simulink model "test_mdl_NI"  (R2018a)
settings: Solver=VariableStepAuto  StartTime=0.0  StopTime=10.0  RelTol=1e-3
(part 11 of 24)

== system test_mdl_NI/Subsystem/IPMA_ADAS/AutoDriveBeam_Data2_Ox3C1 ==
  in_port : Inport
  AdbBrdr2CritLeft_T_Stat : Terminator
  AdbBrdr2CritRigh_T_Stat : Terminator
  AdbBrdr2DistLeft_D_Stat : Terminator
  AdbBrdr2DistRigh_D_Stat : Terminator
  AdbBrdr2Left_An_Rq : Terminator
  AdbBrdr2Low_An_Rq : Terminator
  AdbBrdr2Right_An_Rq : Terminator
  AdbBrdr2Up_An_Rq : Terminator
  AdbIntns2_D_Rq : Terminator
  AdbMde2_D_Rq : Terminator
  bus_selector : BusSelector  OutputSignals=AdbBrdr2CritLeft_T_Stat,AdbBrdr2CritRigh_T_Stat,AdbBrdr2DistLeft_D_Stat,AdbBrdr2DistRigh_D_Stat,AdbBrdr2Left_An_Rq,AdbBrdr2Low_An_Rq,AdbBrdr2Right_An_Rq,AdbBrdr2Up_An_Rq,AdbIntns2_D_Rq,AdbMde2_D_Rq
  wires:
  in_port/1 -> bus_selector/1  "AutoDriveBeam_Data2_Ox3C1"
  bus_selector/1 -> AdbBrdr2CritLeft_T_Stat/1  "<AdbBrdr2CritLeft_T_Stat>"
  bus_selector/2 -> AdbBrdr2CritRigh_T_Stat/1  "<AdbBrdr2CritRigh_T_Stat>"
  bus_selector/3 -> AdbBrdr2DistLeft_D_Stat/1  "<AdbBrdr2DistLeft_D_Stat>"
  bus_selector/4 -> AdbBrdr2DistRigh_D_Stat/1  "<AdbBrdr2DistRigh_D_Stat>"
  bus_selector/5 -> AdbBrdr2Left_An_Rq/1  "<AdbBrdr2Left_An_Rq>"
  bus_selector/6 -> AdbBrdr2Low_An_Rq/1  "<AdbBrdr2Low_An_Rq>"
  bus_selector/7 -> AdbBrdr2Right_An_Rq/1  "<AdbBrdr2Right_An_Rq>"
  bus_selector/8 -> AdbBrdr2Up_An_Rq/1  "<AdbBrdr2Up_An_Rq>"
  bus_selector/9 -> AdbIntns2_D_Rq/1  "<AdbIntns2_D_Rq>"
  bus_selector/10 -> AdbMde2_D_Rq/1  "<AdbMde2_D_Rq>"

== system test_mdl_NI/Subsystem/IPMA_ADAS/AutoDriveBeam_Data3_Ox3C2 ==
  in_port : Inport
  AdbBrdr3CritLeft_T_Stat : Terminator
  AdbBrdr3CritRigh_T_Stat : Terminator
  AdbBrdr3DistLeft_D_Stat : Terminator
  AdbBrdr3DistRigh_D_Stat : Terminator
  AdbBrdr3Left_An_Rq : Terminator
  AdbBrdr3Low_An_Rq : Terminator
  AdbBrdr3Right_An_Rq : Terminator
  AdbBrdr3Up_An_Rq : Terminator
  AdbIntns3_D_Rq : Terminator
  AdbMde3_D_Rq : Terminator
  bus_selector : BusSelector  OutputSignals=AdbBrdr3CritLeft_T_Stat,AdbBrdr3CritRigh_T_Stat,AdbBrdr3DistLeft_D_Stat,AdbBrdr3DistRigh_D_Stat,AdbBrdr3Left_An_Rq,AdbBrdr3Low_An_Rq,AdbBrdr3Right_An_Rq,AdbBrdr3Up_An_Rq,AdbIntns3_D_Rq,AdbMde3_D_Rq
  wires:
  in_port/1 -> bus_selector/1  "AutoDriveBeam_Data3_Ox3C2"
  bus_selector/1 -> AdbBrdr3CritLeft_T_Stat/1  "<AdbBrdr3CritLeft_T_Stat>"
  bus_selector/2 -> AdbBrdr3CritRigh_T_Stat/1  "<AdbBrdr3CritRigh_T_Stat>"
  bus_selector/3 -> AdbBrdr3DistLeft_D_Stat/1  "<AdbBrdr3DistLeft_D_Stat>"
  bus_selector/4 -> AdbBrdr3DistRigh_D_Stat/1  "<AdbBrdr3DistRigh_D_Stat>"
  bus_selector/5 -> AdbBrdr3Left_An_Rq/1  "<AdbBrdr3Left_An_Rq>"
  bus_selector/6 -> AdbBrdr3Low_An_Rq/1  "<AdbBrdr3Low_An_Rq>"
  bus_selector/7 -> AdbBrdr3Right_An_Rq/1  "<AdbBrdr3Right_An_Rq>"
  bus_selector/8 -> AdbBrdr3Up_An_Rq/1  "<AdbBrdr3Up_An_Rq>"
  bus_selector/9 -> AdbIntns3_D_Rq/1  "<AdbIntns3_D_Rq>"
  bus_selector/10 -> AdbMde3_D_Rq/1  "<AdbMde3_D_Rq>"

== system test_mdl_NI/Subsystem/IPMA_ADAS/Bndry_Alert_L_Data_Ox3A1 ==
  in_port : Inport
  BalrChimeLeft_D_Rq : Terminator
  BalrLckLeft_B_Stat : Terminator
  BalrLeft_D_Stat : Terminator
  BalrMdeLeft_D_Stat : Terminator
  BalrMdeSelLeft_B_Stat : Terminator
  BalrSnsLeft_D_Falt : Terminator
  BalrWndwLeft_B_Stat : Terminator
  CamraRearOn_B_RqBalrl : Terminator
  DrLckActv_B_RqBalrl : Terminator
  DrLckCnt_No_ActlBalrl : Terminator
  WndwDrvRear_D_RqBalrl : Terminator
  WndwDrv_D_RqBalrl : Terminator
  WndwPsngrRear_D_RqBalrl : Terminator
  WndwPsngr_D_RqBalrl : Terminator
  bus_selector : BusSelector  OutputSignals=BalrChimeLeft_D_Rq,BalrLckLeft_B_Stat,BalrLeft_D_Stat,BalrMdeLeft_D_Stat,BalrMdeSelLeft_B_Stat,BalrSnsLeft_D_Falt,BalrWndwLeft_B_Stat,CamraRearOn_B_RqBalrl,DrLckActv_B_RqBalrl,DrLckCnt_No_ActlBalrl,WndwDrvRear_D_RqBalrl,WndwDrv_D_RqBalrl,WndwPsngrRear_D_RqBalrl,WndwPsngr_D_RqBalrl
  wires:
  in_port/1 -> bus_selector/1  "Bndry_Alert_L_Data_Ox3A1"
  bus_selector/1 -> BalrChimeLeft_D_Rq/1  "<BalrChimeLeft_D_Rq>"
  bus_selector/2 -> BalrLckLeft_B_Stat/1  "<BalrLckLeft_B_Stat>"
  bus_selector/3 -> BalrLeft_D_Stat/1  "<BalrLeft_D_Stat>"
  bus_selector/4 -> BalrMdeLeft_D_Stat/1  "<BalrMdeLeft_D_Stat>"
  bus_selector/5 -> BalrMdeSelLeft_B_Stat/1  "<BalrMdeSelLeft_B_Stat>"
  bus_selector/6 -> BalrSnsLeft_D_Falt/1  "<BalrSnsLeft_D_Falt>"
  bus_selector/7 -> BalrWndwLeft_B_Stat/1  "<BalrWndwLeft_B_Stat>"
  bus_selector/8 -> CamraRearOn_B_RqBalrl/1  "<CamraRearOn_B_RqBalrl>"
  bus_selector/9 -> DrLckActv_B_RqBalrl/1  "<DrLckActv_B_RqBalrl>"
  bus_selector/10 -> DrLckCnt_No_ActlBalrl/1  "<DrLckCnt_No_ActlBalrl>"
  bus_selector/11 -> WndwDrvRear_D_RqBalrl/1  "<WndwDrvRear_D_RqBalrl>"
  bus_selector/12 -> WndwDrv_D_RqBalrl/1  "<WndwDrv_D_RqBalrl>"
  bus_selector/13 -> WndwPsngrRear_D_RqBalrl/1  "<WndwPsngrRear_D_RqBalrl>"
  bus_selector/14 -> WndwPsngr_D_RqBalrl/1  "<WndwPsngr_D_RqBalrl>"

== system test_mdl_NI/Subsystem/IPMA_ADAS/Bndry_Alert_R_Data_Ox3A2 ==
  in_port : Inport
  BalrChimeRight_D_Rq : Terminator
  BalrLckRight_B_Stat : Terminator
  BalrMdeRight_D_Stat : Terminator
  BalrMdeSelRight_B_Stat : Terminator
  BalrRight_D_Stat : Terminator
  BalrSnsRight_D_Falt : Terminator
  BalrWndwRight_B_Stat : Terminator
  CamraRearOn_B_RqBalrr : Terminator
  DrLckActv_B_RqBalrr : Terminator
  DrLckCnt_No_ActlBalrr : Terminator
  WndwDrvRear_D_RqBalrr : Terminator
  WndwDrv_D_RqBalrr : Terminator
  WndwPsngrRear_D_RqBalrr : Terminator
  WndwPsngr_D_RqBalrr : Terminator
  bus_selector : BusSelector  OutputSignals=BalrChimeRight_D_Rq,BalrLckRight_B_Stat,BalrMdeRight_D_Stat,BalrMdeSelRight_B_Stat,BalrRight_D_Stat,BalrSnsRight_D_Falt,BalrWndwRight_B_Stat,CamraRearOn_B_RqBalrr,DrLckActv_B_RqBalrr,DrLckCnt_No_ActlBalrr,WndwDrvRear_D_RqBalrr,WndwDrv_D_RqBalrr,WndwPsngrRear_D_RqBalrr,WndwPsngr_D_RqBalrr
  wires:
  in_port/1 -> bus_selector/1  "Bndry_Alert_R_Data_Ox3A2"
  bus_selector/1 -> BalrChimeRight_D_Rq/1  "<BalrChimeRight_D_Rq>"
  bus_selector/2 -> BalrLckRight_B_Stat/1  "<BalrLckRight_B_Stat>"
  bus_selector/3 -> BalrMdeRight_D_Stat/1  "<BalrMdeRight_D_Stat>"
  bus_selector/4 -> BalrMdeSelRight_B_Stat/1  "<BalrMdeSelRight_B_Stat>"
  bus_selector/5 -> BalrRight_D_Stat/1  "<BalrRight_D_Stat>"
  bus_selector/6 -> BalrSnsRight_D_Falt/1  "<BalrSnsRight_D_Falt>"
  bus_selector/7 -> BalrWndwRight_B_Stat/1  "<BalrWndwRight_B_Stat>"
  bus_selector/8 -> CamraRearOn_B_RqBalrr/1  "<CamraRearOn_B_RqBalrr>"
  bus_selector/9 -> DrLckActv_B_RqBalrr/1  "<DrLckActv_B_RqBalrr>"
  bus_selector/10 -> DrLckCnt_No_ActlBalrr/1  "<DrLckCnt_No_ActlBalrr>"
  bus_selector/11 -> WndwDrvRear_D_RqBalrr/1  "<WndwDrvRear_D_RqBalrr>"
  bus_selector/12 -> WndwDrv_D_RqBalrr/1  "<WndwDrv_D_RqBalrr>"
  bus_selector/13 -> WndwPsngrRear_D_RqBalrr/1  "<WndwPsngrRear_D_RqBalrr>"
  bus_selector/14 -> WndwPsngr_D_RqBalrr/1  "<WndwPsngr_D_RqBalrr>"

== system test_mdl_NI/Subsystem/IPMA_ADAS/BoundaryAlert_Left_1_Ox4E0 ==
  in_port : Inport
  BalrLeft1CurntX_L_Actl : Terminator
  BalrLeft1CurntY_L_Actl : Terminator
  BalrLeft1Dsply_B_Stat : Terminator
  BalrLeft1Fast_B_Stat : Terminator
  BalrLeft1Prev1X_L_Actl : Terminator
  BalrLeft1Prev1Y_L_Actl : Terminator
  BalrLeft1Prev2X_L_Actl : Terminator
  BalrLeft1Prev2Y_L_Actl : Terminator
  BalrLeft1Prev3X_L_Actl : Terminator
  BalrLeft1Prev3Y_L_Actl : Terminator
  BalrLeft1Threat_D_Stat : Terminator
  bus_selector : BusSelector  OutputSignals=BalrLeft1CurntX_L_Actl,BalrLeft1CurntY_L_Actl,BalrLeft1Dsply_B_Stat,BalrLeft1Fast_B_Stat,BalrLeft1Prev1X_L_Actl,BalrLeft1Prev1Y_L_Actl,BalrLeft1Prev2X_L_Actl,BalrLeft1Prev2Y_L_Actl,BalrLeft1Prev3X_L_Actl,BalrLeft1Prev3Y_L_Actl,BalrLeft1Threat_D_Stat
  wires:
  in_port/1 -> bus_selector/1  "BoundaryAlert_Left_1_Ox4E0"
  bus_selector/1 -> BalrLeft1CurntX_L_Actl/1  "<BalrLeft1CurntX_L_Actl>"
  bus_selector/2 -> BalrLeft1CurntY_L_Actl/1  "<BalrLeft1CurntY_L_Actl>"
  bus_selector/3 -> BalrLeft1Dsply_B_Stat/1  "<BalrLeft1Dsply_B_Stat>"
  bus_selector/4 -> BalrLeft1Fast_B_Stat/1  "<BalrLeft1Fast_B_Stat>"
  bus_selector/5 -> BalrLeft1Prev1X_L_Actl/1  "<BalrLeft1Prev1X_L_Actl>"
  bus_selector/6 -> BalrLeft1Prev1Y_L_Actl/1  "<BalrLeft1Prev1Y_L_Actl>"
  bus_selector/7 -> BalrLeft1Prev2X_L_Actl/1  "<BalrLeft1Prev2X_L_Actl>"
  bus_selector/8 -> BalrLeft1Prev2Y_L_Actl/1  "<BalrLeft1Prev2Y_L_Actl>"
  bus_selector/9 -> BalrLeft1Prev3X_L_Actl/1  "<BalrLeft1Prev3X_L_Actl>"
  bus_selector/10 -> BalrLeft1Prev3Y_L_Actl/1  "<BalrLeft1Prev3Y_L_Actl>"
  bus_selector/11 -> BalrLeft1Threat_D_Stat/1  "<BalrLeft1Threat_D_Stat>"

== system test_mdl_NI/Subsystem/IPMA_ADAS/BoundaryAlert_Left_2_Ox4E1 ==
  in_port : Inport
  BalrLeft2CurntX_L_Actl : Terminator
  BalrLeft2CurntY_L_Actl : Terminator
  BalrLeft2Dsply_B_Stat : Terminator
  BalrLeft2Fast_B_Stat : Terminator
  BalrLeft2Prev1X_L_Actl : Terminator
  BalrLeft2Prev1Y_L_Actl : Terminator
  BalrLeft2Prev2X_L_Actl : Terminator
  BalrLeft2Prev2Y_L_Actl : Terminator
  BalrLeft2Prev3X_L_Actl : Terminator
  BalrLeft2Prev3Y_L_Actl : Terminator
  BalrLeft2Threat_D_Stat : Terminator
  bus_selector : BusSelector  OutputSignals=BalrLeft2CurntX_L_Actl,BalrLeft2CurntY_L_Actl,BalrLeft2Dsply_B_Stat,BalrLeft2Fast_B_Stat,BalrLeft2Prev1X_L_Actl,BalrLeft2Prev1Y_L_Actl,BalrLeft2Prev2X_L_Actl,BalrLeft2Prev2Y_L_Actl,BalrLeft2Prev3X_L_Actl,BalrLeft2Prev3Y_L_Actl,BalrLeft2Threat_D_Stat
  wires:
  in_port/1 -> bus_selector/1  "BoundaryAlert_Left_2_Ox4E1"
  bus_selector/1 -> BalrLeft2CurntX_L_Actl/1  "<BalrLeft2CurntX_L_Actl>"
  bus_selector/2 -> BalrLeft2CurntY_L_Actl/1  "<BalrLeft2CurntY_L_Actl>"
  bus_selector/3 -> BalrLeft2Dsply_B_Stat/1  "<BalrLeft2Dsply_B_Stat>"
  bus_selector/4 -> BalrLeft2Fast_B_Stat/1  "<BalrLeft2Fast_B_Stat>"
  bus_selector/5 -> BalrLeft2Prev1X_L_Actl/1  "<BalrLeft2Prev1X_L_Actl>"
  bus_selector/6 -> BalrLeft2Prev1Y_L_Actl/1  "<BalrLeft2Prev1Y_L_Actl>"
  bus_selector/7 -> BalrLeft2Prev2X_L_Actl/1  "<BalrLeft2Prev2X_L_Actl>"
  bus_selector/8 -> BalrLeft2Prev2Y_L_Actl/1  "<BalrLeft2Prev2Y_L_Actl>"
  bus_selector/9 -> BalrLeft2Prev3X_L_Actl/1  "<BalrLeft2Prev3X_L_Actl>"
  bus_selector/10 -> BalrLeft2Prev3Y_L_Actl/1  "<BalrLeft2Prev3Y_L_Actl>"
  bus_selector/11 -> BalrLeft2Threat_D_Stat/1  "<BalrLeft2Threat_D_Stat>"

== system test_mdl_NI/Subsystem/IPMA_ADAS/BoundaryAlert_Left_3_Ox4E2 ==
  in_port : Inport
  BalrLeft3CurntX_L_Actl : Terminator
  BalrLeft3CurntY_L_Actl : Terminator
  BalrLeft3Dsply_B_Stat : Terminator
  BalrLeft3Fast_B_Stat : Terminator
  BalrLeft3Prev1X_L_Actl : Terminator
  BalrLeft3Prev1Y_L_Actl : Terminator
  BalrLeft3Prev2X_L_Actl : Terminator
  BalrLeft3Prev2Y_L_Actl : Terminator
  BalrLeft3Prev3X_L_Actl : Terminator
  BalrLeft3Prev3Y_L_Actl : Terminator
  BalrLeft3Threat_D_Stat : Terminator
  bus_selector : BusSelector  OutputSignals=BalrLeft3CurntX_L_Actl,BalrLeft3CurntY_L_Actl,BalrLeft3Dsply_B_Stat,BalrLeft3Fast_B_Stat,BalrLeft3Prev1X_L_Actl,BalrLeft3Prev1Y_L_Actl,BalrLeft3Prev2X_L_Actl,BalrLeft3Prev2Y_L_Actl,BalrLeft3Prev3X_L_Actl,BalrLeft3Prev3Y_L_Actl,BalrLeft3Threat_D_Stat
  wires:
  in_port/1 -> bus_selector/1  "BoundaryAlert_Left_3_Ox4E2"
  bus_selector/1 -> BalrLeft3CurntX_L_Actl/1  "<BalrLeft3CurntX_L_Actl>"
  bus_selector/2 -> BalrLeft3CurntY_L_Actl/1  "<BalrLeft3CurntY_L_Actl>"
  bus_selector/3 -> BalrLeft3Dsply_B_Stat/1  "<BalrLeft3Dsply_B_Stat>"
  bus_selector/4 -> BalrLeft3Fast_B_Stat/1  "<BalrLeft3Fast_B_Stat>"
  bus_selector/5 -> BalrLeft3Prev1X_L_Actl/1  "<BalrLeft3Prev1X_L_Actl>"
  bus_selector/6 -> BalrLeft3Prev1Y_L_Actl/1  "<BalrLeft3Prev1Y_L_Actl>"
  bus_selector/7 -> BalrLeft3Prev2X_L_Actl/1  "<BalrLeft3Prev2X_L_Actl>"
  bus_selector/8 -> BalrLeft3Prev2Y_L_Actl/1  "<BalrLeft3Prev2Y_L_Actl>"
  bus_selector/9 -> BalrLeft3Prev3X_L_Actl/1  "<BalrLeft3Prev3X_L_Actl>"
  bus_selector/10 -> BalrLeft3Prev3Y_L_Actl/1  "<BalrLeft3Prev3Y_L_Actl>"
  bus_selector/11 -> BalrLeft3Threat_D_Stat/1  "<BalrLeft3Threat_D_Stat>"

== system test_mdl_NI/Subsystem/IPMA_ADAS/BoundaryAlert_Left_4_Ox4E3 ==
  in_port : Inport
  BalrLeft4CurntX_L_Actl : Terminator
  BalrLeft4CurntY_L_Actl : Terminator
  BalrLeft4Dsply_B_Stat : Terminator
  BalrLeft4Fast_B_Stat : Terminator
  BalrLeft4Prev1X_L_Actl : Terminator
  BalrLeft4Prev1Y_L_Actl : Terminator
  BalrLeft4Prev2X_L_Actl : Terminator
  BalrLeft4Prev2Y_L_Actl : Terminator
  BalrLeft4Prev3X_L_Actl : Terminator
  BalrLeft4Prev3Y_L_Actl : Terminator
  BalrLeft4Threat_D_Stat : Terminator
  bus_selector : BusSelector  OutputSignals=BalrLeft4CurntX_L_Actl,BalrLeft4CurntY_L_Actl,BalrLeft4Dsply_B_Stat,BalrLeft4Fast_B_Stat,BalrLeft4Prev1X_L_Actl,BalrLeft4Prev1Y_L_Actl,BalrLeft4Prev2X_L_Actl,BalrLeft4Prev2Y_L_Actl,BalrLeft4Prev3X_L_Actl,BalrLeft4Prev3Y_L_Actl,BalrLeft4Threat_D_Stat
  wires:
  in_port/1 -> bus_selector/1  "BoundaryAlert_Left_4_Ox4E3"
  bus_selector/1 -> BalrLeft4CurntX_L_Actl/1  "<BalrLeft4CurntX_L_Actl>"
  bus_selector/2 -> BalrLeft4CurntY_L_Actl/1  "<BalrLeft4CurntY_L_Actl>"
  bus_selector/3 -> BalrLeft4Dsply_B_Stat/1  "<BalrLeft4Dsply_B_Stat>"
  bus_selector/4 -> BalrLeft4Fast_B_Stat/1  "<BalrLeft4Fast_B_Stat>"
  bus_selector/5 -> BalrLeft4Prev1X_L_Actl/1  "<BalrLeft4Prev1X_L_Actl>"
  bus_selector/6 -> BalrLeft4Prev1Y_L_Actl/1  "<BalrLeft4Prev1Y_L_Actl>"
  bus_selector/7 -> BalrLeft4Prev2X_L_Actl/1  "<BalrLeft4Prev2X_L_Actl>"
  bus_selector/8 -> BalrLeft4Prev2Y_L_Actl/1  "<BalrLeft4Prev2Y_L_Actl>"
  bus_selector/9 -> BalrLeft4Prev3X_L_Actl/1  "<BalrLeft4Prev3X_L_Actl>"
  bus_selector/10 -> BalrLeft4Prev3Y_L_Actl/1  "<BalrLeft4Prev3Y_L_Actl>"
  bus_selector/11 -> BalrLeft4Threat_D_Stat/1  "<BalrLeft4Threat_D_Stat>"

== system test_mdl_NI/Subsystem/IPMA_ADAS/BoundaryAlert_Right_1_Ox4E4 ==
  in_port : Inport
  BalrRight1CurntX_L_Actl : Terminator
  BalrRight1CurntY_L_Actl : Terminator
  BalrRight1Dsply_B_Stat : Terminator
  BalrRight1Fast_B_Stat : Terminator
  BalrRight1Prev1X_L_Actl : Terminator
  BalrRight1Prev1Y_L_Actl : Terminator
  BalrRight1Prev2X_L_Actl : Terminator
  BalrRight1Prev2Y_L_Actl : Terminator
  BalrRight1Prev3X_L_Actl : Terminator
  BalrRight1Prev3Y_L_Actl : Terminator
  BalrRight1Threat_D_Stat : Terminator
  bus_selector : BusSelector  OutputSignals=BalrRight1CurntX_L_Actl,BalrRight1CurntY_L_Actl,BalrRight1Dsply_B_Stat,BalrRight1Fast_B_Stat,BalrRight1Prev1X_L_Actl,BalrRight1Prev1Y_L_Actl,BalrRight1Prev2X_L_Actl,BalrRight1Prev2Y_L_Actl,BalrRight1Prev3X_L_Actl,BalrRight1Prev3Y_L_Actl,BalrRight1Threat_D_Stat
  wires:
  in_port/1 -> bus_selector/1  "BoundaryAlert_Right_1_Ox4E4"
  bus_selector/1 -> BalrRight1CurntX_L_Actl/1  "<BalrRight1CurntX_L_Actl>"
  bus_selector/2 -> BalrRight1CurntY_L_Actl/1  "<BalrRight1CurntY_L_Actl>"
  bus_selector/3 -> BalrRight1Dsply_B_Stat/1  "<BalrRight1Dsply_B_Stat>"
  bus_selector/4 -> BalrRight1Fast_B_Stat/1  "<BalrRight1Fast_B_Stat>"
  bus_selector/5 -> BalrRight1Prev1X_L_Actl/1  "<BalrRight1Prev1X_L_Actl>"
  bus_selector/6 -> BalrRight1Prev1Y_L_Actl/1  "<BalrRight1Prev1Y_L_Actl>"
  bus_selector/7 -> BalrRight1Prev2X_L_Actl/1  "<BalrRight1Prev2X_L_Actl>"
  bus_selector/8 -> BalrRight1Prev2Y_L_Actl/1  "<BalrRight1Prev2Y_L_Actl>"
  bus_selector/9 -> BalrRight1Prev3X_L_Actl/1  "<BalrRight1Prev3X_L_Actl>"
  bus_selector/10 -> BalrRight1Prev3Y_L_Actl/1  "<BalrRight1Prev3Y_L_Actl>"
  bus_selector/11 -> BalrRight1Threat_D_Stat/1  "<BalrRight1Threat_D_Stat>"

== system test_mdl_NI/Subsystem/IPMA_ADAS/BoundaryAlert_Right_2_Ox4E5 ==
  in_port : Inport
  BalrRight2CurntX_L_Actl : Terminator
  BalrRight2CurntY_L_Actl : Terminator
  BalrRight2Dsply_B_Stat : Terminator
  BalrRight2Fast_B_Stat : Terminator
  BalrRight2Prev1X_L_Actl : Terminator
  BalrRight2Prev1Y_L_Actl : Terminator
  BalrRight2Prev2X_L_Actl : Terminator
  BalrRight2Prev2Y_L_Actl : Terminator
  BalrRight2Prev3X_L_Actl : Terminator
  BalrRight2Prev3Y_L_Actl : Terminator
  BalrRight2Threat_D_Stat : Terminator
  bus_selector : BusSelector  OutputSignals=BalrRight2CurntX_L_Actl,BalrRight2CurntY_L_Actl,BalrRight2Dsply_B_Stat,BalrRight2Fast_B_Stat,BalrRight2Prev1X_L_Actl,BalrRight2Prev1Y_L_Actl,BalrRight2Prev2X_L_Actl,BalrRight2Prev2Y_L_Actl,BalrRight2Prev3X_L_Actl,BalrRight2Prev3Y_L_Actl,BalrRight2Threat_D_Stat
  wires:
  in_port/1 -> bus_selector/1  "BoundaryAlert_Right_2_Ox4E5"
  bus_selector/1 -> BalrRight2CurntX_L_Actl/1  "<BalrRight2CurntX_L_Actl>"
  bus_selector/2 -> BalrRight2CurntY_L_Actl/1  "<BalrRight2CurntY_L_Actl>"
  bus_selector/3 -> BalrRight2Dsply_B_Stat/1  "<BalrRight2Dsply_B_Stat>"
  bus_selector/4 -> BalrRight2Fast_B_Stat/1  "<BalrRight2Fast_B_Stat>"
  bus_selector/5 -> BalrRight2Prev1X_L_Actl/1  "<BalrRight2Prev1X_L_Actl>"
  bus_selector/6 -> BalrRight2Prev1Y_L_Actl/1  "<BalrRight2Prev1Y_L_Actl>"
  bus_selector/7 -> BalrRight2Prev2X_L_Actl/1  "<BalrRight2Prev2X_L_Actl>"
  bus_selector/8 -> BalrRight2Prev2Y_L_Actl/1  "<BalrRight2Prev2Y_L_Actl>"
  bus_selector/9 -> BalrRight2Prev3X_L_Actl/1  "<BalrRight2Prev3X_L_Actl>"
  bus_selector/10 -> BalrRight2Prev3Y_L_Actl/1  "<BalrRight2Prev3Y_L_Actl>"
  bus_selector/11 -> BalrRight2Threat_D_Stat/1  "<BalrRight2Threat_D_Stat>"

== system test_mdl_NI/Subsystem/IPMA_ADAS/BoundaryAlert_Right_3_Ox4E6 ==
  in_port : Inport
  BalrRight3CurntX_L_Actl : Terminator
  BalrRight3CurntY_L_Actl : Terminator
  BalrRight3Dsply_B_Stat : Terminator
  BalrRight3Fast_B_Stat : Terminator
  BalrRight3Prev1X_L_Actl : Terminator
  BalrRight3Prev1Y_L_Actl : Terminator
  BalrRight3Prev2X_L_Actl : Terminator
  BalrRight3Prev2Y_L_Actl : Terminator
  BalrRight3Prev3X_L_Actl : Terminator
  BalrRight3Prev3Y_L_Actl : Terminator
  BalrRight3Threat_D_Stat : Terminator
  bus_selector : BusSelector  OutputSignals=BalrRight3CurntX_L_Actl,BalrRight3CurntY_L_Actl,BalrRight3Dsply_B_Stat,BalrRight3Fast_B_Stat,BalrRight3Prev1X_L_Actl,BalrRight3Prev1Y_L_Actl,BalrRight3Prev2X_L_Actl,BalrRight3Prev2Y_L_Actl,BalrRight3Prev3X_L_Actl,BalrRight3Prev3Y_L_Actl,BalrRight3Threat_D_Stat
  wires:
  in_port/1 -> bus_selector/1  "BoundaryAlert_Right_3_Ox4E6"
  bus_selector/1 -> BalrRight3CurntX_L_Actl/1  "<BalrRight3CurntX_L_Actl>"
  bus_selector/2 -> BalrRight3CurntY_L_Actl/1  "<BalrRight3CurntY_L_Actl>"
  bus_selector/3 -> BalrRight3Dsply_B_Stat/1  "<BalrRight3Dsply_B_Stat>"
  bus_selector/4 -> BalrRight3Fast_B_Stat/1  "<BalrRight3Fast_B_Stat>"
  bus_selector/5 -> BalrRight3Prev1X_L_Actl/1  "<BalrRight3Prev1X_L_Actl>"
  bus_selector/6 -> BalrRight3Prev1Y_L_Actl/1  "<BalrRight3Prev1Y_L_Actl>"
  bus_selector/7 -> BalrRight3Prev2X_L_Actl/1  "<BalrRight3Prev2X_L_Actl>"
  bus_selector/8 -> BalrRight3Prev2Y_L_Actl/1  "<BalrRight3Prev2Y_L_Actl>"
  bus_selector/9 -> BalrRight3Prev3X_L_Actl/1  "<BalrRight3Prev3X_L_Actl>"
  bus_selector/10 -> BalrRight3Prev3Y_L_Actl/1  "<BalrRight3Prev3Y_L_Actl>"
  bus_selector/11 -> BalrRight3Threat_D_Stat/1  "<BalrRight3Threat_D_Stat>"

== system test_mdl_NI/Subsystem/IPMA_ADAS/BoundaryAlert_Right_4_Ox4E7 ==
  in_port : Inport
  BalrRight4CurntX_L_Actl : Terminator
  BalrRight4CurntY_L_Actl : Terminator
  BalrRight4Dsply_B_Stat : Terminator
  BalrRight4Fast_B_Stat : Terminator
  BalrRight4Prev1X_L_Actl : Terminator
  BalrRight4Prev1Y_L_Actl : Terminator
  BalrRight4Prev2X_L_Actl : Terminator
  BalrRight4Prev2Y_L_Actl : Terminator
  BalrRight4Prev3X_L_Actl : Terminator
  BalrRight4Prev3Y_L_Actl : Terminator
  BalrRight4Threat_D_Stat : Terminator
  bus_selector : BusSelector  OutputSignals=BalrRight4CurntX_L_Actl,BalrRight4CurntY_L_Actl,BalrRight4Dsply_B_Stat,BalrRight4Fast_B_Stat,BalrRight4Prev1X_L_Actl,BalrRight4Prev1Y_L_Actl,BalrRight4Prev2X_L_Actl,BalrRight4Prev2Y_L_Actl,BalrRight4Prev3X_L_Actl,BalrRight4Prev3Y_L_Actl,BalrRight4Threat_D_Stat
  wires:
  in_port/1 -> bus_selector/1  "BoundaryAlert_Right_4_Ox4E7"
  bus_selector/1 -> BalrRight4CurntX_L_Actl/1  "<BalrRight4CurntX_L_Actl>"
  bus_selector/2 -> BalrRight4CurntY_L_Actl/1  "<BalrRight4CurntY_L_Actl>"
  bus_selector/3 -> BalrRight4Dsply_B_Stat/1  "<BalrRight4Dsply_B_Stat>"
  bus_selector/4 -> BalrRight4Fast_B_Stat/1  "<BalrRight4Fast_B_Stat>"
  bus_selector/5 -> BalrRight4Prev1X_L_Actl/1  "<BalrRight4Prev1X_L_Actl>"
  bus_selector/6 -> BalrRight4Prev1Y_L_Actl/1  "<BalrRight4Prev1Y_L_Actl>"
  bus_selector/7 -> BalrRight4Prev2X_L_Actl/1  "<BalrRight4Prev2X_L_Actl>"
  bus_selector/8 -> BalrRight4Prev2Y_L_Actl/1  "<BalrRight4Prev2Y_L_Actl>"
  bus_selector/9 -> BalrRight4Prev3X_L_Actl/1  "<BalrRight4Prev3X_L_Actl>"
  bus_selector/10 -> BalrRight4Prev3Y_L_Actl/1  "<BalrRight4Prev3Y_L_Actl>"
  bus_selector/11 -> BalrRight4Threat_D_Stat/1  "<BalrRight4Threat_D_Stat>"

== system test_mdl_NI/Subsystem/IPMA_ADAS/GlareFreeBeam_Ox3D5 ==
  in_port : Inport
  AdbBeam_D_Rq : Terminator
  AdbBrdrBottom_An_Rq : Terminator
  AdbBrdrLeft_An_Rq : Terminator
  AdbBrdrLeft_L_Stat : Terminator
  AdbBrdrRight_An_Rq : Terminator
  AdbBrdrRight_L_Stat : Terminator
  AdbBrdrTop_An_Rq : Terminator
  AdbRamping_T_Rq : Terminator
  bus_selector : BusSelector  OutputSignals=AdbBeam_D_Rq,AdbBrdrBottom_An_Rq,AdbBrdrLeft_An_Rq,AdbBrdrLeft_L_Stat,AdbBrdrRight_An_Rq,AdbBrdrRight_L_Stat,AdbBrdrTop_An_Rq,AdbRamping_T_Rq
  wires:
  in_port/1 -> bus_selector/1  "GlareFreeBeam_Ox3D5"
  bus_selector/1 -> AdbBeam_D_Rq/1  "<AdbBeam_D_Rq>"
  bus_selector/2 -> AdbBrdrBottom_An_Rq/1  "<AdbBrdrBottom_An_Rq>"
  bus_selector/3 -> AdbBrdrLeft_An_Rq/1  "<AdbBrdrLeft_An_Rq>"
  bus_selector/4 -> AdbBrdrLeft_L_Stat/1  "<AdbBrdrLeft_L_Stat>"
  bus_selector/5 -> AdbBrdrRight_An_Rq/1  "<AdbBrdrRight_An_Rq>"
  bus_selector/6 -> AdbBrdrRight_L_Stat/1  "<AdbBrdrRight_L_Stat>"
  bus_selector/7 -> AdbBrdrTop_An_Rq/1  "<AdbBrdrTop_An_Rq>"
  bus_selector/8 -> AdbRamping_T_Rq/1  "<AdbRamping_T_Rq>"

== system test_mdl_NI/Subsystem/IPMA_ADAS/IPMA_Data2_Ox3D9 ==
  in_port : Inport
  AdbDividedRoad_B_Stat : Terminator
  AdbDrvSide_B_Stat : Terminator
  DasAlrtInfo_D_Dsply : Terminator
  IaccVLimUnit_D_Rq : Terminator
  IaccVLim_D_Rq : Terminator
  IsaVLimUnit_D_Rq : Terminator
  IsaVLim_D_Rq : Terminator
  LcwaMsgTxt_D_Stat : Terminator
  LdwChime_B_Rq : Terminator
  LongCtrlEnbl_D_Rq : Terminator
  SblmPedCrossScnr_B_Stat : Terminator
  SblmRndAbtScnr_B_Stat : Terminator
  SblmStopScnr_B_Stat : Terminator
  SblmYieldScnr_B_Stat : Terminator
  TsrRegionTxt_D_Stat : Terminator
  bus_selector : BusSelector  OutputSignals=AdbDividedRoad_B_Stat,AdbDrvSide_B_Stat,DasAlrtInfo_D_Dsply,IaccVLimUnit_D_Rq,IaccVLim_D_Rq,IsaVLimUnit_D_Rq,IsaVLim_D_Rq,LcwaMsgTxt_D_Stat,LdwChime_B_Rq,LongCtrlEnbl_D_Rq,SblmPedCrossScnr_B_Stat,SblmRndAbtScnr_B_Stat,SblmStopScnr_B_Stat,SblmYieldScnr_B_Stat,TsrRegionTxt_D_Stat
  wires:
  in_port/1 -> bus_selector/1  "IPMA_Data2_Ox3D9"
  bus_selector/1 -> AdbDividedRoad_B_Stat/1  "<AdbDividedRoad_B_Stat>"
  bus_selector/2 -> AdbDrvSide_B_Stat/1  "<AdbDrvSide_B_Stat>"
  bus_selector/3 -> DasAlrtInfo_D_Dsply/1  "<DasAlrtInfo_D_Dsply>"
  bus_selector/4 -> IaccVLimUnit_D_Rq/1  "<IaccVLimUnit_D_Rq>"
  bus_selector/5 -> IaccVLim_D_Rq/1  "<IaccVLim_D_Rq>"
  bus_selector/6 -> IsaVLimUnit_D_Rq/1  "<IsaVLimUnit_D_Rq>"
  bus_selector/7 -> IsaVLim_D_Rq/1  "<IsaVLim_D_Rq>"
  bus_selector/8 -> LcwaMsgTxt_D_Stat/1  "<LcwaMsgTxt_D_Stat>"
  bus_selector/9 -> LdwChime_B_Rq/1  "<LdwChime_B_Rq>"
  bus_selector/10 -> LongCtrlEnbl_D_Rq/1  "<LongCtrlEnbl_D_Rq>"
  bus_selector/11 -> SblmPedCrossScnr_B_Stat/1  "<SblmPedCrossScnr_B_Stat>"
  bus_selector/12 -> SblmRndAbtScnr_B_Stat/1  "<SblmRndAbtScnr_B_Stat>"
  bus_selector/13 -> SblmStopScnr_B_Stat/1  "<SblmStopScnr_B_Stat>"
  bus_selector/14 -> SblmYieldScnr_B_Stat/1  "<SblmYieldScnr_B_Stat>"
  bus_selector/15 -> TsrRegionTxt_D_Stat/1  "<TsrRegionTxt_D_Stat>"

== system test_mdl_NI/Subsystem/IPMA_ADAS/IPMA_Data3_Ox3F2 ==
  in_port : Inport
  AdbUrbanArea_B_Stat : Terminator
  CbdblActv_B_RqAdas : Terminator
  LightCurv_NoRate_Actl : Terminator
  LightCurv_No_Actl : Terminator
  LightPathOffst_L_Actl : Terminator
  LightPath_An_Actl : Terminator
  LightRng_L_Max : Terminator
  MbdblActv_B_RqAdas : Terminator
  bus_selector : BusSelector  OutputSignals=AdbUrbanArea_B_Stat,CbdblActv_B_RqAdas,LightCurv_NoRate_Actl,LightCurv_No_Actl,LightPathOffst_L_Actl,LightPath_An_Actl,LightRng_L_Max,MbdblActv_B_RqAdas
  wires:
  in_port/1 -> bus_selector/1  "IPMA_Data3_Ox3F2"
  bus_selector/1 -> AdbUrbanArea_B_Stat/1  "<AdbUrbanArea_B_Stat>"
  bus_selector/2 -> CbdblActv_B_RqAdas/1  "<CbdblActv_B_RqAdas>"
  bus_selector/3 -> LightCurv_NoRate_Actl/1  "<LightCurv_NoRate_Actl>"
  bus_selector/4 -> LightCurv_No_Actl/1  "<LightCurv_No_Actl>"
  bus_selector/5 -> LightPathOffst_L_Actl/1  "<LightPathOffst_L_Actl>"
  bus_selector/6 -> LightPath_An_Actl/1  "<LightPath_An_Actl>"
  bus_selector/7 -> LightRng_L_Max/1  "<LightRng_L_Max>"
  bus_selector/8 -> MbdblActv_B_RqAdas/1  "<MbdblActv_B_RqAdas>"

== system test_mdl_NI/Subsystem/IPMA_ADAS/IPMA_Data4_Ox3AF ==
  in_port : Inport
  AdasLcDistToObj_L_Actl : Terminator
  VehVActlAdas_D_Qf : Terminator
  Veh_V_ActlAdas : Terminator
  Veh_V_RqLsc : Terminator
  bus_selector : BusSelector  OutputSignals=AdasLcDistToObj_L_Actl,VehVActlAdas_D_Qf,Veh_V_ActlAdas,Veh_V_RqLsc
  wires:
  in_port/1 -> bus_selector/1  "IPMA_Data4_Ox3AF"
  bus_selector/1 -> AdasLcDistToObj_L_Actl/1  "<AdasLcDistToObj_L_Actl>"
  bus_selector/2 -> VehVActlAdas_D_Qf/1  "<VehVActlAdas_D_Qf>"
  bus_selector/3 -> Veh_V_ActlAdas/1  "<Veh_V_ActlAdas>"
  bus_selector/4 -> Veh_V_RqLsc/1  "<Veh_V_RqLsc>"

== system test_mdl_NI/Subsystem/IPMA_ADAS/IPMA_Data_Ox3D8 ==
  in_port : Inport
  AhbHiBeam_D_Rq : Terminator
  AhbcRampingV_D_Rq : Terminator
  CamraDefog_B_Req : Terminator
  CamraStats_D_Dsply : Terminator
  DasAlrtLvl_D_Dsply : Terminator
  DasStats_D_Dsply : Terminator
  DasWarn_D_Dsply : Terminator
  FeatConfigIpmaActl : Terminator
  FeatNoIpmaActl : Terminator
  LaActvStats_D_Dsply : Terminator
  LaDenyStats_B_Dsply : Terminator
  LaHandsOff_D_Dsply : Terminator
  PersIndexIpma_D_Actl : Terminator
  bus_selector : BusSelector  OutputSignals=AhbHiBeam_D_Rq,AhbcRampingV_D_Rq,CamraDefog_B_Req,CamraStats_D_Dsply,DasAlrtLvl_D_Dsply,DasStats_D_Dsply,DasWarn_D_Dsply,FeatConfigIpmaActl,FeatNoIpmaActl,LaActvStats_D_Dsply,LaDenyStats_B_Dsply,LaHandsOff_D_Dsply,PersIndexIpma_D_Actl
  wires:
  in_port/1 -> bus_selector/1  "IPMA_Data_Ox3D8"
  bus_selector/1 -> AhbHiBeam_D_Rq/1  "<AhbHiBeam_D_Rq>"
  bus_selector/2 -> AhbcRampingV_D_Rq/1  "<AhbcRampingV_D_Rq>"
  bus_selector/3 -> CamraDefog_B_Req/1  "<CamraDefog_B_Req>"
  bus_selector/4 -> CamraStats_D_Dsply/1  "<CamraStats_D_Dsply>"
  bus_selector/5 -> DasAlrtLvl_D_Dsply/1  "<DasAlrtLvl_D_Dsply>"
  bus_selector/6 -> DasStats_D_Dsply/1  "<DasStats_D_Dsply>"
  bus_selector/7 -> DasWarn_D_Dsply/1  "<DasWarn_D_Dsply>"
  bus_selector/8 -> FeatConfigIpmaActl/1  "<FeatConfigIpmaActl>"
  bus_selector/9 -> FeatNoIpmaActl/1  "<FeatNoIpmaActl>"
  bus_selector/10 -> LaActvStats_D_Dsply/1  "<LaActvStats_D_Dsply>"
  bus_selector/11 -> LaDenyStats_B_Dsply/1  "<LaDenyStats_B_Dsply>"
  bus_selector/12 -> LaHandsOff_D_Dsply/1  "<LaHandsOff_D_Dsply>"
  bus_selector/13 -> PersIndexIpma_D_Actl/1  "<PersIndexIpma_D_Actl>"

== system test_mdl_NI/Subsystem/IPMA_ADAS/Image_Processing_Data_Ox451 ==
  in_port : Inport
  BrkDecel_B_RqRba : Terminator
  BrkEnbl_B_RqRba : Terminator
  CamraFrntStat_D_Stat : Terminator
  RbaAlrt_D_Dsply : Terminator
  RbaMnu_D_Rq : Terminator
  RbaMsg_D_Rq : Terminator
  Rba_D_Stat : Terminator
  TrlrAidEnbl_D_RqAdas : Terminator
  TrlrAidSwtchLamp_B_Rq : Terminator
  TrlrHitchChime_D_Rq : Terminator
  TrlrHitchIcon_D_Rq : Terminator
  TrlrHitchLamp_D_Rq2 : Terminator
  TrlrHitchMsgTxt_D_Rq : Terminator
  TrlrRvrseEnbl_D2_Stat : Terminator
  TrlrRvrseMsgTxt_D2_Rq : Terminator
  bus_selector : BusSelector  OutputSignals=BrkDecel_B_RqRba,BrkEnbl_B_RqRba,CamraFrntStat_D_Stat,RbaAlrt_D_Dsply,RbaMnu_D_Rq,RbaMsg_D_Rq,Rba_D_Stat,TrlrAidEnbl_D_RqAdas,TrlrAidSwtchLamp_B_Rq,TrlrHitchChime_D_Rq,TrlrHitchIcon_D_Rq,TrlrHitchLamp_D_Rq2,TrlrHitchMsgTxt_D_Rq,TrlrRvrseEnbl_D2_Stat,TrlrRvrseMsgTxt_D2_Rq
  wires:
  in_port/1 -> bus_selector/1  "Image_Processing_Data_Ox451"
  bus_selector/1 -> BrkDecel_B_RqRba/1  "<BrkDecel_B_RqRba>"
  bus_selector/2 -> BrkEnbl_B_RqRba/1  "<BrkEnbl_B_RqRba>"
  bus_selector/3 -> CamraFrntStat_D_Stat/1  "<CamraFrntStat_D_Stat>"
  bus_selector/4 -> RbaAlrt_D_Dsply/1  "<RbaAlrt_D_Dsply>"
  bus_selector/5 -> RbaMnu_D_Rq/1  "<RbaMnu_D_Rq>"
  bus_selector/6 -> RbaMsg_D_Rq/1  "<RbaMsg_D_Rq>"
  bus_selector/7 -> Rba_D_Stat/1  "<Rba_D_Stat>"
  bus_selector/8 -> TrlrAidEnbl_D_RqAdas/1  "<TrlrAidEnbl_D_RqAdas>"
  bus_selector/9 -> TrlrAidSwtchLamp_B_Rq/1  "<TrlrAidSwtchLamp_B_Rq>"
  bus_selector/10 -> TrlrHitchChime_D_Rq/1  "<TrlrHitchChime_D_Rq>"
  bus_selector/11 -> TrlrHitchIcon_D_Rq/1  "<TrlrHitchIcon_D_Rq>"
  bus_selector/12 -> TrlrHitchLamp_D_Rq2/1  "<TrlrHitchLamp_D_Rq2>"
  bus_selector/13 -> TrlrHitchMsgTxt_D_Rq/1  "<TrlrHitchMsgTxt_D_Rq>"
  bus_selector/14 -> TrlrRvrseEnbl_D2_Stat/1  "<TrlrRvrseEnbl_D2_Stat>"
  bus_selector/15 -> TrlrRvrseMsgTxt_D2_Rq/1  "<TrlrRvrseMsgTxt_D2_Rq>"

== system test_mdl_NI/Subsystem/IPMA_ADAS/Lane_Assist_Data1_Ox3CA ==
  in_port : Inport
  LaCurvature_No_Calc : Terminator
  LaRampType_B_Req : Terminator
  LaRefAng_No_Req : Terminator
  LdwActvIntns_D_Req : Terminator
  LdwActvStats_D_Req : Terminator
  LkaActvStats_D2_Req : Terminator
  LkaDrvOvrrd_D_Rq : Terminator
  bus_selector : BusSelector  OutputSignals=LaCurvature_No_Calc,LaRampType_B_Req,LaRefAng_No_Req,LdwActvIntns_D_Req,LdwActvStats_D_Req,LkaActvStats_D2_Req,LkaDrvOvrrd_D_Rq
  wires:
  in_port/1 -> bus_selector/1  "Lane_Assist_Data1_Ox3CA"
  bus_selector/1 -> LaCurvature_No_Calc/1  "<LaCurvature_No_Calc>"
  bus_selector/2 -> LaRampType_B_Req/1  "<LaRampType_B_Req>"
  bus_selector/3 -> LaRefAng_No_Req/1  "<LaRefAng_No_Req>"
  bus_selector/4 -> LdwActvIntns_D_Req/1  "<LdwActvIntns_D_Req>"
  bus_selector/5 -> LdwActvStats_D_Req/1  "<LdwActvStats_D_Req>"
  bus_selector/6 -> LkaActvStats_D2_Req/1  "<LkaActvStats_D2_Req>"
  bus_selector/7 -> LkaDrvOvrrd_D_Rq/1  "<LkaDrvOvrrd_D_Rq>"

== system test_mdl_NI/Subsystem/IPMA_ADAS/LateralMotionControl2_Ox3D6 ==
  in_port : Inport
  HandsOffCnfm_B_Rq : Terminator
  LatCtlCrv_NoRate2_Actl : Terminator
  LatCtlCurv_No_Actl : Terminator
  LatCtlPathOffst_L_Actl : Terminator
  LatCtlPath_An_Actl : Terminator
  LatCtlPath_No_Cnt : Terminator
  LatCtlPath_No_Cs : Terminator
  LatCtlPrecision_D_Rq : Terminator
  LatCtlRampType_D_Rq : Terminator
  LatCtl_D2_Rq : Terminator
  bus_selector : BusSelector  OutputSignals=HandsOffCnfm_B_Rq,LatCtlCrv_NoRate2_Actl,LatCtlCurv_No_Actl,LatCtlPathOffst_L_Actl,LatCtlPath_An_Actl,LatCtlPath_No_Cnt,LatCtlPath_No_Cs,LatCtlPrecision_D_Rq,LatCtlRampType_D_Rq,LatCtl_D2_Rq
  wires:
  in_port/1 -> bus_selector/1  "LateralMotionControl2_Ox3D6"
  bus_selector/1 -> HandsOffCnfm_B_Rq/1  "<HandsOffCnfm_B_Rq>"
  bus_selector/2 -> LatCtlCrv_NoRate2_Actl/1  "<LatCtlCrv_NoRate2_Actl>"
  bus_selector/3 -> LatCtlCurv_No_Actl/1  "<LatCtlCurv_No_Actl>"
  bus_selector/4 -> LatCtlPathOffst_L_Actl/1  "<LatCtlPathOffst_L_Actl>"
  bus_selector/5 -> LatCtlPath_An_Actl/1  "<LatCtlPath_An_Actl>"
  bus_selector/6 -> LatCtlPath_No_Cnt/1  "<LatCtlPath_No_Cnt>"
  bus_selector/7 -> LatCtlPath_No_Cs/1  "<LatCtlPath_No_Cs>"
  bus_selector/8 -> LatCtlPrecision_D_Rq/1  "<LatCtlPrecision_D_Rq>"
  bus_selector/9 -> LatCtlRampType_D_Rq/1  "<LatCtlRampType_D_Rq>"
  bus_selector/10 -> LatCtl_D2_Rq/1  "<LatCtl_D2_Rq>"

== system test_mdl_NI/Subsystem/IPMA_ADAS/LateralMotionControl_Ox3D3 ==
  in_port : Inport
  HandsOffCnfm_B_Rq : Terminator
  LatCtlCurv_NoRate_Actl : Terminator
  LatCtlCurv_No_Actl : Terminator
  LatCtlPathOffst_L_Actl : Terminator
  LatCtlPath_An_Actl : Terminator
  LatCtlPrecision_D_Rq : Terminator
  LatCtlRampType_D_Rq : Terminator
  LatCtlRng_L_Max : Terminator
  LatCtl_D_Rq : Terminator
  bus_selector : BusSelector  OutputSignals=HandsOffCnfm_B_Rq,LatCtlCurv_NoRate_Actl,LatCtlCurv_No_Actl,LatCtlPathOffst_L_Actl,LatCtlPath_An_Actl,LatCtlPrecision_D_Rq,LatCtlRampType_D_Rq,LatCtlRng_L_Max,LatCtl_D_Rq
  wires:
  in_port/1 -> bus_selector/1  "LateralMotionControl_Ox3D3"
  bus_selector/1 -> HandsOffCnfm_B_Rq/1  "<HandsOffCnfm_B_Rq>"
  bus_selector/2 -> LatCtlCurv_NoRate_Actl/1  "<LatCtlCurv_NoRate_Actl>"
  bus_selector/3 -> LatCtlCurv_No_Actl/1  "<LatCtlCurv_No_Actl>"
  bus_selector/4 -> LatCtlPathOffst_L_Actl/1  "<LatCtlPathOffst_L_Actl>"
  bus_selector/5 -> LatCtlPath_An_Actl/1  "<LatCtlPath_An_Actl>"
  bus_selector/6 -> LatCtlPrecision_D_Rq/1  "<LatCtlPrecision_D_Rq>"
  bus_selector/7 -> LatCtlRampType_D_Rq/1  "<LatCtlRampType_D_Rq>"
  bus_selector/8 -> LatCtlRng_L_Max/1  "<LatCtlRng_L_Max>"
  bus_selector/9 -> LatCtl_D_Rq/1  "<LatCtl_D_Rq>"

== system test_mdl_NI/Subsystem/IPMA_ADAS/OTAPhysCCMtoGWM_ECG_Ox1B936015 ==
  in_port : Inport
  OTAPhysCCMtoGWM_ECG : Terminator
  bus_selector : BusSelector  OutputSignals=OTAPhysCCMtoGWM_ECG
  wires:
  in_port/1 -> bus_selector/1  "OTAPhysCCMtoGWM_ECG_Ox1B936015"
  bus_selector/1 -> OTAPhysCCMtoGWM_ECG/1  "<OTAPhysCCMtoGWM_ECG>"

== system test_mdl_NI/Subsystem/IPMA_ADAS/OTAPhysIPMAtoGWM_ECG_Ox1B936021 ==
  in_port : Inport
  OTAPhysIPMAtoGWM_ECG : Terminator
  bus_selector : BusSelector  OutputSignals=OTAPhysIPMAtoGWM_ECG
  wires:
  in_port/1 -> bus_selector/1  "OTAPhysIPMAtoGWM_ECG_Ox1B936021"
  bus_selector/1 -> OTAPhysIPMAtoGWM_ECG/1  "<OTAPhysIPMAtoGWM_ECG>"

== system test_mdl_NI/Subsystem/IPMA_ADAS/OTAPhysSODCMCtoGWM_ECG_Ox1B936045 ==
  in_port : Inport
  OTAPhysSODCMCtoGWM_ECG : Terminator
  bus_selector : BusSelector  OutputSignals=OTAPhysSODCMCtoGWM_ECG
  wires:
  in_port/1 -> bus_selector/1  "OTAPhysSODCMCtoGWM_ECG_Ox1B936045"
  bus_selector/1 -> OTAPhysSODCMCtoGWM_ECG/1  "<OTAPhysSODCMCtoGWM_ECG>"

== system test_mdl_NI/Subsystem/IPMA_ADAS/OTAPhysSODCMDtoGWM_ECG_Ox1B936046 ==
  in_port : Inport
  OTAPhysSODCMDtoGWM_ECG : Terminator
  bus_selector : BusSelector  OutputSignals=OTAPhysSODCMDtoGWM_ECG
  wires:
  in_port/1 -> bus_selector/1  "OTAPhysSODCMDtoGWM_ECG_Ox1B936046"
  bus_selector/1 -> OTAPhysSODCMDtoGWM_ECG/1  "<OTAPhysSODCMDtoGWM_ECG>"

== system test_mdl_NI/Subsystem/IPMA_ADAS/OTAPhysSODLtoGWM_ECG_Ox1B936062 ==
  in_port : Inport
  OTAPhysSODLtoGWM_ECG : Terminator
  bus_selector : BusSelector  OutputSignals=OTAPhysSODLtoGWM_ECG
  wires:
  in_port/1 -> bus_selector/1  "OTAPhysSODLtoGWM_ECG_Ox1B936062"
  bus_selector/1 -> OTAPhysSODLtoGWM_ECG/1  "<OTAPhysSODLtoGWM_ECG>"

== system test_mdl_NI/Subsystem/IPMA_ADAS/OTAPhysSODRtoGWM_ECG_Ox1B936063 ==
  in_port : Inport
  OTAPhysSODRtoGWM_ECG : Terminator
  bus_selector : BusSelector  OutputSignals=OTAPhysSODRtoGWM_ECG
  wires:
  in_port/1 -> bus_selector/1  "OTAPhysSODRtoGWM_ECG_Ox1B936063"
  bus_selector/1 -> OTAPhysSODRtoGWM_ECG/1  "<OTAPhysSODRtoGWM_ECG>"

== system test_mdl_NI/Subsystem/IPMA_ADAS/PARSEDPhysCCMtoGWM_ECG_Ox1BA36015 ==
  in_port : Inport
  PARSEDPhysCCMtoGWM_ECG : Terminator
  bus_selector : BusSelector  OutputSignals=PARSEDPhysCCMtoGWM_ECG
  wires:
  in_port/1 -> bus_selector/1  "PARSEDPhysCCMtoGWM_ECG_Ox1BA36015"
  bus_selector/1 -> PARSEDPhysCCMtoGWM_ECG/1  "<PARSEDPhysCCMtoGWM_ECG>"

== system test_mdl_NI/Subsystem/IPMA_ADAS/PARSEDPhysIPMAtoGWM_ECG_Ox1BA36021 ==
  in_port : Inport
  PARSEDPhysIPMAtoGWM_ECG : Terminator
  bus_selector : BusSelector  OutputSignals=PARSEDPhysIPMAtoGWM_ECG
  wires:
  in_port/1 -> bus_selector/1  "PARSEDPhysIPMAtoGWM_ECG_Ox1BA36021"
  bus_selector/1 -> PARSEDPhysIPMAtoGWM_ECG/1  "<PARSEDPhysIPMAtoGWM_ECG>"

== system test_mdl_NI/Subsystem/IPMA_ADAS/PARSEDPhysSODCMCtoGWM_ECG_Ox1BA36045 ==
  in_port : Inport
  PARSEDPhysSODCMCtoGWM_ECG : Terminator
  bus_selector : BusSelector  OutputSignals=PARSEDPhysSODCMCtoGWM_ECG
  wires:
  in_port/1 -> bus_selector/1  "PARSEDPhysSODCMCtoGWM_ECG_Ox1BA36045"
  bus_selector/1 -> PARSEDPhysSODCMCtoGWM_ECG/1  "<PARSEDPhysSODCMCtoGWM_ECG>"

== system test_mdl_NI/Subsystem/IPMA_ADAS/PARSEDPhysSODCMDtoGWM_ECG_Ox1BA36046 ==
  in_port : Inport
  PARSEDPhysSODCMDtoGWM_ECG : Terminator
  bus_selector : BusSelector  OutputSignals=PARSEDPhysSODCMDtoGWM_ECG
  wires:
  in_port/1 -> bus_selector/1  "PARSEDPhysSODCMDtoGWM_ECG_Ox1BA36046"
  bus_selector/1 -> PARSEDPhysSODCMDtoGWM_ECG/1  "<PARSEDPhysSODCMDtoGWM_ECG>"

== system test_mdl_NI/Subsystem/IPMA_ADAS/PARSEDPhysSODLtoGWM_ECG_Ox1BA36062 ==
  in_port : Inport
  PARSEDPhysSODLtoGWM_ECG : Terminator
  bus_selector : BusSelector  OutputSignals=PARSEDPhysSODLtoGWM_ECG
  wires:
  in_port/1 -> bus_selector/1  "PARSEDPhysSODLtoGWM_ECG_Ox1BA36062"
  bus_selector/1 -> PARSEDPhysSODLtoGWM_ECG/1  "<PARSEDPhysSODLtoGWM_ECG>"

== system test_mdl_NI/Subsystem/IPMA_ADAS/PARSEDPhysSODRtoGWM_ECG_Ox1BA36063 ==
  in_port : Inport
  PARSEDPhysSODRtoGWM_ECG : Terminator
  bus_selector : BusSelector  OutputSignals=PARSEDPhysSODRtoGWM_ECG
  wires:
  in_port/1 -> bus_selector/1  "PARSEDPhysSODRtoGWM_ECG_Ox1BA36063"
  bus_selector/1 -> PARSEDPhysSODRtoGWM_ECG/1  "<PARSEDPhysSODRtoGWM_ECG>"

== system test_mdl_NI/Subsystem/IPMA_ADAS/PARSEDPushCCMtoGWM_ECG_Ox1BB36015 ==
  in_port : Inport
  PARSEDPhysCCM2toGWM_ECG : Terminator
  bus_selector : BusSelector  OutputSignals=PARSEDPhysCCM2toGWM_ECG
  wires:
  in_port/1 -> bus_selector/1  "PARSEDPushCCMtoGWM_ECG_Ox1BB36015"
  bus_selector/1 -> PARSEDPhysCCM2toGWM_ECG/1  "<PARSEDPhysCCM2toGWM_ECG>"

== system test_mdl_NI/Subsystem/IPMA_ADAS/PARSEDPushIPMAtoGWM_ECG_Ox1BB36021 ==
  in_port : Inport
  PARSEDPhysIPMA2toGWM_ECG : Terminator
  bus_selector : BusSelector  OutputSignals=PARSEDPhysIPMA2toGWM_ECG
  wires:
  in_port/1 -> bus_selector/1  "PARSEDPushIPMAtoGWM_ECG_Ox1BB36021"
  bus_selector/1 -> PARSEDPhysIPMA2toGWM_ECG/1  "<PARSEDPhysIPMA2toGWM_ECG>"

== system test_mdl_NI/Subsystem/IPMA_ADAS/PARSEDPushSODCMCtoGWM_Ox1BB36045 ==
  in_port : Inport
  PARSEDPhysSODCMC2toGWM_ECG : Terminator
  bus_selector : BusSelector  OutputSignals=PARSEDPhysSODCMC2toGWM_ECG
  wires:
  in_port/1 -> bus_selector/1  "PARSEDPushSODCMCtoGWM_Ox1BB36045"
  bus_selector/1 -> PARSEDPhysSODCMC2toGWM_ECG/1  "<PARSEDPhysSODCMC2toGWM_ECG>"

== system test_mdl_NI/Subsystem/IPMA_ADAS/PARSEDPushSODCMDtoGWM_Ox1BB36046 ==
  in_port : Inport
  PARSEDPhysSODCMD2toGWM_ECG : Terminator
  bus_selector : BusSelector  OutputSignals=PARSEDPhysSODCMD2toGWM_ECG
  wires:
  in_port/1 -> bus_selector/1  "PARSEDPushSODCMDtoGWM_Ox1BB36046"
  bus_selector/1 -> PARSEDPhysSODCMD2toGWM_ECG/1  "<PARSEDPhysSODCMD2toGWM_ECG>"

== system test_mdl_NI/Subsystem/IPMA_ADAS/PARSEDPushSODLtoGWM_ECG_Ox1BB36062 ==
  in_port : Inport
  PARSEDPhysSODL2toGWM_ECG : Terminator
  bus_selector : BusSelector  OutputSignals=PARSEDPhysSODL2toGWM_ECG
  wires:
  in_port/1 -> bus_selector/1  "PARSEDPushSODLtoGWM_ECG_Ox1BB36062"
  bus_selector/1 -> PARSEDPhysSODL2toGWM_ECG/1  "<PARSEDPhysSODL2toGWM_ECG>"

== system test_mdl_NI/Subsystem/IPMA_ADAS/PARSEDPushSODRtoGWM_ECG_Ox1BB36063 ==
  in_port : Inport
  PARSEDPhysSODR2toGWM_ECG : Terminator
  bus_selector : BusSelector  OutputSignals=PARSEDPhysSODR2toGWM_ECG
  wires:
  in_port/1 -> bus_selector/1  "PARSEDPushSODRtoGWM_ECG_Ox1BB36063"
  bus_selector/1 -> PARSEDPhysSODR2toGWM_ECG/1  "<PARSEDPhysSODR2toGWM_ECG>"

== system test_mdl_NI/Subsystem/IPMA_ADAS/ParkAid_Aud_Warn_Stat2_Ox3AB ==
  in_port : Inport
  ApaBrk_A_Rq : Terminator
  ApaBrk_D_Rq : Terminator
  ApaLongCtrlEnbl_D_Rq : Terminator
  PrkAidChime_D_Stat : Terminator
  PrkAidFront_D_Stat : Terminator
  PrkAidLamp_D_Rq : Terminator
  PrkAidRear_D_Stat : Terminator
  PrkAidSnsRlCntr_D_Stat : Terminator
  PrkAidSnsRlCrnr_D_Stat : Terminator
  PrkAidSnsRrCntr_D_Stat : Terminator
  PrkAidSnsRrCrnr_D_Stat : Terminator
  PrkAid_D_Falt : Terminator
  SidePrkSnsL3_D_Stat : Terminator
  SidePrkSnsL4_D_Stat : Terminator
  SidePrkSnsR3_D_Stat : Terminator
  SidePrkSnsR4_D_Stat : Terminator
  bus_selector : BusSelector  OutputSignals=ApaBrk_A_Rq,ApaBrk_D_Rq,ApaLongCtrlEnbl_D_Rq,PrkAidChime_D_Stat,PrkAidFront_D_Stat,PrkAidLamp_D_Rq,PrkAidRear_D_Stat,PrkAidSnsRlCntr_D_Stat,PrkAidSnsRlCrnr_D_Stat,PrkAidSnsRrCntr_D_Stat,PrkAidSnsRrCrnr_D_Stat,PrkAid_D_Falt,SidePrkSnsL3_D_Stat,SidePrkSnsL4_D_Stat,SidePrkSnsR3_D_Stat,SidePrkSnsR4_D_Stat
  wires:
  in_port/1 -> bus_selector/1  "ParkAid_Aud_Warn_Stat2_Ox3AB"
  bus_selector/1 -> ApaBrk_A_Rq/1  "<ApaBrk_A_Rq>"
  bus_selector/2 -> ApaBrk_D_Rq/1  "<ApaBrk_D_Rq>"
  bus_selector/3 -> ApaLongCtrlEnbl_D_Rq/1  "<ApaLongCtrlEnbl_D_Rq>"
  bus_selector/4 -> PrkAidChime_D_Stat/1  "<PrkAidChime_D_Stat>"
  bus_selector/5 -> PrkAidFront_D_Stat/1  "<PrkAidFront_D_Stat>"
  bus_selector/6 -> PrkAidLamp_D_Rq/1  "<PrkAidLamp_D_Rq>"
  bus_selector/7 -> PrkAidRear_D_Stat/1  "<PrkAidRear_D_Stat>"
  bus_selector/8 -> PrkAidSnsRlCntr_D_Stat/1  "<PrkAidSnsRlCntr_D_Stat>"
  bus_selector/9 -> PrkAidSnsRlCrnr_D_Stat/1  "<PrkAidSnsRlCrnr_D_Stat>"
  bus_selector/10 -> PrkAidSnsRrCntr_D_Stat/1  "<PrkAidSnsRrCntr_D_Stat>"
  bus_selector/11 -> PrkAidSnsRrCrnr_D_Stat/1  "<PrkAidSnsRrCrnr_D_Stat>"
  bus_selector/12 -> PrkAid_D_Falt/1  "<PrkAid_D_Falt>"
  bus_selector/13 -> SidePrkSnsL3_D_Stat/1  "<SidePrkSnsL3_D_Stat>"
  bus_selector/14 -> SidePrkSnsL4_D_Stat/1  "<SidePrkSnsL4_D_Stat>"
  bus_selector/15 -> SidePrkSnsR3_D_Stat/1  "<SidePrkSnsR3_D_Stat>"
  bus_selector/16 -> SidePrkSnsR4_D_Stat/1  "<SidePrkSnsR4_D_Stat>"

== system test_mdl_NI/Subsystem/IPMA_ADAS/ParkAid_Aud_Warn_Stat_Ox3AA ==
  in_port : Inport
  ApaActvSd_D_Actl : Terminator
  ApaMde_D_Avail : Terminator
  ApaMde_D_Stat : Terminator
  FpaChime_D_Rq : Terminator
  PrkAidAudioMute_B_Rq : Terminator
  PrkAidMsgTxt_D_Rq : Terminator
  PrkAidSnsFlCntr_D_Stat : Terminator
  PrkAidSnsFlCrnr_D_Stat : Terminator
  PrkAidSnsFrCntr_D_Stat : Terminator
  PrkAidSnsFrCrnr_D_Stat : Terminator
  PrkAidSwtch_B_Stat : Terminator
  PrkBrkEl_B_RqFap : Terminator
  RpaChime_D_Rq : Terminator
  SidePrkSnsL1_D_Stat : Terminator
  SidePrkSnsL2_D_Stat : Terminator
  SidePrkSnsR1_D_Stat : Terminator
  SidePrkSnsR2_D_Stat : Terminator
  bus_selector : BusSelector  OutputSignals=ApaActvSd_D_Actl,ApaMde_D_Avail,ApaMde_D_Stat,FpaChime_D_Rq,PrkAidAudioMute_B_Rq,PrkAidMsgTxt_D_Rq,PrkAidSnsFlCntr_D_Stat,PrkAidSnsFlCrnr_D_Stat,PrkAidSnsFrCntr_D_Stat,PrkAidSnsFrCrnr_D_Stat,PrkAidSwtch_B_Stat,PrkBrkEl_B_RqFap,RpaChime_D_Rq,SidePrkSnsL1_D_Stat,SidePrkSnsL2_D_Stat,SidePrkSnsR1_D_Stat,SidePrkSnsR2_D_Stat
  wires:
  in_port/1 -> bus_selector/1  "ParkAid_Aud_Warn_Stat_Ox3AA"
  bus_selector/1 -> ApaActvSd_D_Actl/1  "<ApaActvSd_D_Actl>"
  bus_selector/2 -> ApaMde_D_Avail/1  "<ApaMde_D_Avail>"
  bus_selector/3 -> ApaMde_D_Stat/1  "<ApaMde_D_Stat>"
  bus_selector/4 -> FpaChime_D_Rq/1  "<FpaChime_D_Rq>"
  bus_selector/5 -> PrkAidAudioMute_B_Rq/1  "<PrkAidAudioMute_B_Rq>"
  bus_selector/6 -> PrkAidMsgTxt_D_Rq/1  "<PrkAidMsgTxt_D_Rq>"
  bus_selector/7 -> PrkAidSnsFlCntr_D_Stat/1  "<PrkAidSnsFlCntr_D_Stat>"
  bus_selector/8 -> PrkAidSnsFlCrnr_D_Stat/1  "<PrkAidSnsFlCrnr_D_Stat>"
  bus_selector/9 -> PrkAidSnsFrCntr_D_Stat/1  "<PrkAidSnsFrCntr_D_Stat>"
  bus_selector/10 -> PrkAidSnsFrCrnr_D_Stat/1  "<PrkAidSnsFrCrnr_D_Stat>"
  bus_selector/11 -> PrkAidSwtch_B_Stat/1  "<PrkAidSwtch_B_Stat>"
  bus_selector/12 -> PrkBrkEl_B_RqFap/1  "<PrkBrkEl_B_RqFap>"
  bus_selector/13 -> RpaChime_D_Rq/1  "<RpaChime_D_Rq>"
  bus_selector/14 -> SidePrkSnsL1_D_Stat/1  "<SidePrkSnsL1_D_Stat>"
  bus_selector/15 -> SidePrkSnsL2_D_Stat/1  "<SidePrkSnsL2_D_Stat>"
  bus_selector/16 -> SidePrkSnsR1_D_Stat/1  "<SidePrkSnsR1_D_Stat>"
  bus_selector/17 -> SidePrkSnsR2_D_Stat/1  "<SidePrkSnsR2_D_Stat>"

== system test_mdl_NI/Subsystem/IPMA_ADAS/ParkAid_Data2_Ox3AE ==
  in_port : Inport
  PrkAidAcsyFront_D_Stat : Terminator
  PrkAidAcsyRear_D_Stat : Terminator
  PrkAidDrvDir_D_Stat : Terminator
  PrkAidRdiusLeft_L_Dsply : Terminator
  PrkAidRdiusRight_L_Dsply : Terminator
  bus_selector : BusSelector  OutputSignals=PrkAidAcsyFront_D_Stat,PrkAidAcsyRear_D_Stat,PrkAidDrvDir_D_Stat,PrkAidRdiusLeft_L_Dsply,PrkAidRdiusRight_L_Dsply
  wires:
  in_port/1 -> bus_selector/1  "ParkAid_Data2_Ox3AE"
  bus_selector/1 -> PrkAidAcsyFront_D_Stat/1  "<PrkAidAcsyFront_D_Stat>"
  bus_selector/2 -> PrkAidAcsyRear_D_Stat/1  "<PrkAidAcsyRear_D_Stat>"
  bus_selector/3 -> PrkAidDrvDir_D_Stat/1  "<PrkAidDrvDir_D_Stat>"
  bus_selector/4 -> PrkAidRdiusLeft_L_Dsply/1  "<PrkAidRdiusLeft_L_Dsply>"
  bus_selector/5 -> PrkAidRdiusRight_L_Dsply/1  "<PrkAidRdiusRight_L_Dsply>"

== system test_mdl_NI/Subsystem/IPMA_ADAS/ParkAid_Data_2_Ox3A9 ==
  in_port : Inport
  FapLcDistToObj_L_Actl : Terminator
  TrnRngDRqFap_No_Cnt : Terminator
  TrnRngDRqFap_No_Cs : Terminator
  TrnRng_D_RqFap : Terminator
  Veh_V_RqFap : Terminator
  bus_selector : BusSelector  OutputSignals=FapLcDistToObj_L_Actl,TrnRngDRqFap_No_Cnt,TrnRngDRqFap_No_Cs,TrnRng_D_RqFap,Veh_V_RqFap
  wires:
  in_port/1 -> bus_selector/1  "ParkAid_Data_2_Ox3A9"
  bus_selector/1 -> FapLcDistToObj_L_Actl/1  "<FapLcDistToObj_L_Actl>"
  bus_selector/2 -> TrnRngDRqFap_No_Cnt/1  "<TrnRngDRqFap_No_Cnt>"
  bus_selector/3 -> TrnRngDRqFap_No_Cs/1  "<TrnRngDRqFap_No_Cs>"
  bus_selector/4 -> TrnRng_D_RqFap/1  "<TrnRng_D_RqFap>"
  bus_selector/5 -> Veh_V_RqFap/1  "<Veh_V_RqFap>"

== system test_mdl_NI/Subsystem/IPMA_ADAS/ParkAid_Data_Ox3A8 ==
  in_port : Inport
  ApaAcsy_D_RqDrv : Terminator
  ApaActvSide2_D_Stat : Terminator
  ApaButtnPrssd_B_Stat : Terminator
  ApaChime_D_Rq : Terminator
  ApaGearShif_D_RqDrv : Terminator
  ApaLongCtl_D_RqDrv : Terminator
  ApaMsgTxt_D_Rq : Terminator
  ApaScan_D_Stat : Terminator
  ApaSelPoa_D_Stat : Terminator
  ApaSelPpa_D_Stat : Terminator
  ApaSelSapp_D_Stat : Terminator
  ApaSteScanMde_D_Stat : Terminator
  ApaSteWhl_D_RqDrv : Terminator
  ApaSys_D_Stat : Terminator
  ApaTrgtDist_D_Stat : Terminator
  EPASExtAngleStatReq : Terminator
  ExtSteeringAngleReq2 : Terminator
  SAPPStatusCoding : Terminator
  bus_selector : BusSelector  OutputSignals=ApaAcsy_D_RqDrv,ApaActvSide2_D_Stat,ApaButtnPrssd_B_Stat,ApaChime_D_Rq,ApaGearShif_D_RqDrv,ApaLongCtl_D_RqDrv,ApaMsgTxt_D_Rq,ApaScan_D_Stat,ApaSelPoa_D_Stat,ApaSelPpa_D_Stat,ApaSelSapp_D_Stat,ApaSteScanMde_D_Stat,ApaSteWhl_D_RqDrv,ApaSys_D_Stat,ApaTrgtDist_D_Stat,EPASExtAngleStatReq,ExtSteeringAngleReq2,SAPPStatusCoding
  wires:
  in_port/1 -> bus_selector/1  "ParkAid_Data_Ox3A8"
  bus_selector/1 -> ApaAcsy_D_RqDrv/1  "<ApaAcsy_D_RqDrv>"
  bus_selector/2 -> ApaActvSide2_D_Stat/1  "<ApaActvSide2_D_Stat>"
  bus_selector/3 -> ApaButtnPrssd_B_Stat/1  "<ApaButtnPrssd_B_Stat>"
  bus_selector/4 -> ApaChime_D_Rq/1  "<ApaChime_D_Rq>"
  bus_selector/5 -> ApaGearShif_D_RqDrv/1  "<ApaGearShif_D_RqDrv>"
  bus_selector/6 -> ApaLongCtl_D_RqDrv/1  "<ApaLongCtl_D_RqDrv>"
  bus_selector/7 -> ApaMsgTxt_D_Rq/1  "<ApaMsgTxt_D_Rq>"
  bus_selector/8 -> ApaScan_D_Stat/1  "<ApaScan_D_Stat>"
  bus_selector/9 -> ApaSelPoa_D_Stat/1  "<ApaSelPoa_D_Stat>"
  bus_selector/10 -> ApaSelPpa_D_Stat/1  "<ApaSelPpa_D_Stat>"
  bus_selector/11 -> ApaSelSapp_D_Stat/1  "<ApaSelSapp_D_Stat>"
  bus_selector/12 -> ApaSteScanMde_D_Stat/1  "<ApaSteScanMde_D_Stat>"
  bus_selector/13 -> ApaSteWhl_D_RqDrv/1  "<ApaSteWhl_D_RqDrv>"
  bus_selector/14 -> ApaSys_D_Stat/1  "<ApaSys_D_Stat>"
  bus_selector/15 -> ApaTrgtDist_D_Stat/1  "<ApaTrgtDist_D_Stat>"
  bus_selector/16 -> EPASExtAngleStatReq/1  "<EPASExtAngleStatReq>"
  bus_selector/17 -> ExtSteeringAngleReq2/1  "<ExtSteeringAngleReq2>"
  bus_selector/18 -> SAPPStatusCoding/1  "<SAPPStatusCoding>"

== system test_mdl_NI/Subsystem/IPMA_ADAS/Personality_CCM_Data_Ox3E5 ==
  in_port : Inport
  FeatConfigCcmActl : Terminator
  FeatNoCcmActl : Terminator
  PersIndexCcm_D_Actl : Terminator
  bus_selector : BusSelector  OutputSignals=FeatConfigCcmActl,FeatNoCcmActl,PersIndexCcm_D_Actl
  wires:
  in_port/1 -> bus_selector/1  "Personality_CCM_Data_Ox3E5"
  bus_selector/1 -> FeatConfigCcmActl/1  "<FeatConfigCcmActl>"
  bus_selector/2 -> FeatNoCcmActl/1  "<FeatNoCcmActl>"
  bus_selector/3 -> PersIndexCcm_D_Actl/1  "<PersIndexCcm_D_Actl>"

== system test_mdl_NI/Subsystem/IPMA_ADAS/Personality_IPMB_Data_Ox3EE ==
  in_port : Inport
  FeatConfigIpmbActl : Terminator
  FeatNoIpmbActl : Terminator
  PersIndexIpmb_D_Actl : Terminator
  bus_selector : BusSelector  OutputSignals=FeatConfigIpmbActl,FeatNoIpmbActl,PersIndexIpmb_D_Actl
  wires:
  in_port/1 -> bus_selector/1  "Personality_IPMB_Data_Ox3EE"
  bus_selector/1 -> FeatConfigIpmbActl/1  "<FeatConfigIpmbActl>"
  bus_selector/2 -> FeatNoIpmbActl/1  "<FeatNoIpmbActl>"
  bus_selector/3 -> PersIndexIpmb_D_Actl/1  "<PersIndexIpmb_D_Actl>"
